simulink model "EEEUI (1)"  (R2024b)
settings: Solver=VariableStepAuto  StartTime=0.0  StopTime=10.0  RelTol=1e-3
libraries: spsBreakerLib x6, spsThreePhaseSourceLib x3, spsGroundLib x2, spsThreePhaseParallelRLCLoadLib x2, spsThreePhaseTransformer12TerminalsLib x2, spsThreePhaseSeriesRLCLoadLib x1, spsThreePhaseVIMeasurementLib x1, spsThreePhaseBreakerLib x1, spsThreePhaseFaultLib x1
settings Model: Creator=praji

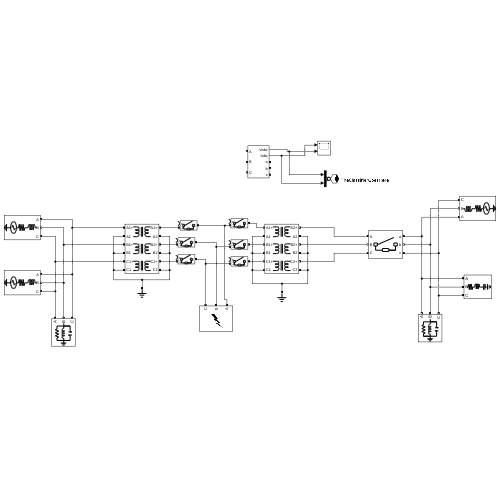
[thumbnail: Simulink's stored preview of the top-level diagram]
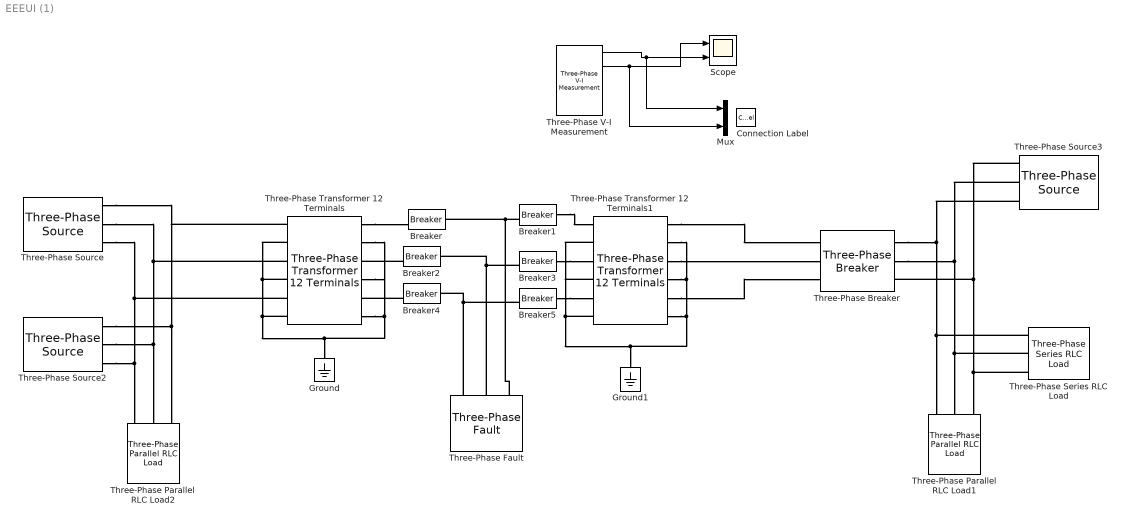
== system EEEUI (1) ==
  Breaker{,1..5} (6 alike) : spsBreakerLib/Breaker  InitialState=0  SwitchingTimes="[1/60  5/60]"  External=on  BreakerResistance=0.01  SnubberResistance=1e6  SnubberCapacitance=inf  Measurements=None  MoreParameters=on  NoBreakLoop=off
  Connection Label : ConnectionLabel  Label=TheClassifierGoesHere
  Ground : spsGroundLib/Ground  LConnTagsString=a
  Ground1 : spsGroundLib/Ground  LConnTagsString=a
  Mux : Mux  Inputs=2
  Scope : Scope  NumInputPorts=2
  Three-Phase Parallel RLC Load1 : spsThreePhaseParallelRLCLoadLib/Three-Phase Parallel RLC Load  LConnTagsString=A|B|C  Configuration=Y (grounded)  NominalVoltage=1000  Vabc=[1e3 1e3 1e3]  Vabcp=[1e3 1e3 1e3]  NominalFrequency=60  UnbalancedPower=off  ActivePower=10e3  InductivePower=100  CapacitivePower=100  Pabc=[10e3 9e3 11e3]  QLabc=[100 90 110]  QCabc=[100 90 110]  Pabcp=[10e3 9e3 11e3]  QLabcp=[100 90 110]  QCabcp=[100 90 110]  Measurements=None  LoadType=constant Z
  Three-Phase Parallel RLC Load2 : spsThreePhaseParallelRLCLoadLib/Three-Phase Parallel RLC Load  LConnTagsString=A|B|C  Configuration=Y (grounded)  NominalVoltage=1000  Vabc=[1e3 1e3 1e3]  Vabcp=[1e3 1e3 1e3]  NominalFrequency=60  UnbalancedPower=off  ActivePower=10e3  InductivePower=100  CapacitivePower=100  Pabc=[10e3 9e3 11e3]  QLabc=[100 90 110]  QCabc=[100 90 110]  Pabcp=[10e3 9e3 11e3]  QLabcp=[100 90 110]  QCabcp=[100 90 110]  Measurements=None  LoadType=constant Z
  Three-Phase Series RLC Load : spsThreePhaseSeriesRLCLoadLib/Three-Phase Series RLC Load  LConnTagsString=A|B|C  Configuration=Y (grounded)  NominalVoltage=1000  Vabc=[1e3 1e3 1e3]  Vabcp=[1e3 1e3 1e3]  NominalFrequency=60  UnbalancedPower=off  ActivePower=10e3  InductivePower=100  CapacitivePower=100  Pabc=[10e3 9e3 11e3]  QLabc=[100 90 110]  QCabc=[100 90 110]  Pabcp=[10e3 9e3 11e3]  QLabcp=[100 90 110]  QCabcp=[100 90 110]  Measurements=None  LoadType=constant Z
  Three-Phase V-I Measurement : spsThreePhaseVIMeasurementLib/Three-Phase V-I Measurement  VoltageMeasurement=phase-to-ground  SetLabelV=off  LabelV=Vabc  Vpu=off  VpuLL=off  CurrentMeasurement=yes  SetLabelI=off  LabelI=Iabc  Ipu=off  Pbase=100e6  Vbase=500e3  OutputType=Complex  PhasorSimulation=off  PSBequivalent=0
  Three-Phase Breaker : spsThreePhaseBreakerLib/Three-Phase Breaker  InitialState=open  SwitchA=on  SwitchB=on  SwitchC=on  SwitchTimes="[1/60  5/60]"  External=off  BreakerResistance=0.01  SnubberResistance=1e6  SnubberCapacitance=inf  Measurements=None
  Three-Phase Fault : spsThreePhaseFaultLib/Three-Phase Fault  InitialStates=0  FaultA=on  FaultB=on  FaultC=on  GroundFault=on  SwitchTimes="[1/60  5/60]"  External=off  SwitchStatus=NaN  FaultResistance=0.001  GroundResistance=0.01  SnubberResistance=1e6  SnubberCapacitance=inf  Measurements=None
  Three-Phase Source : spsThreePhaseSourceLib/Three-Phase Source  InternalConnection=Yg  VoltagePhases=off  Voltage=25e3  PhaseAngle=0  Voltage_phases=[25e3 25e3 25e3]/sqrt(3)  PhaseAngles_phases=[0 -120 +120]  Frequency=60  NonIdealSource=on  SpecifyImpedance=off  Resistance=0.8929  Inductance=16.58e-3  ShortCircuitLevel=100e6  BaseVoltage=25e3  XRratio=7  BusType=swing  Pref=10e3  Qref=0  Prefabc=[10e3, 10e3, 10e3]  Qrefabc=[0, 0, 0]  Qmin=-inf  Qmax=inf
  Three-Phase Source2 : spsThreePhaseSourceLib/Three-Phase Source  InternalConnection=Yg  VoltagePhases=off  Voltage=25e3  PhaseAngle=0  Voltage_phases=[25e3 25e3 25e3]/sqrt(3)  PhaseAngles_phases=[0 -120 +120]  Frequency=60  NonIdealSource=on  SpecifyImpedance=off  Resistance=0.8929  Inductance=16.58e-3  ShortCircuitLevel=100e6  BaseVoltage=25e3  XRratio=7  BusType=swing  Pref=10e3  Qref=0  Prefabc=[10e3, 10e3, 10e3]  Qrefabc=[0, 0, 0]  Qmin=-inf  Qmax=inf
  Three-Phase Source3 : spsThreePhaseSourceLib/Three-Phase Source  InternalConnection=Yg  VoltagePhases=off  Voltage=25e3  PhaseAngle=0  Voltage_phases=[25e3 25e3 25e3]/sqrt(3)  PhaseAngles_phases=[0 -120 +120]  Frequency=60  NonIdealSource=on  SpecifyImpedance=off  Resistance=0.8929  Inductance=16.58e-3  ShortCircuitLevel=100e6  BaseVoltage=25e3  XRratio=7  BusType=swing  Pref=10e3  Qref=0  Prefabc=[10e3, 10e3, 10e3]  Qrefabc=[0, 0, 0]  Qmin=-inf  Qmax=inf
  Three-Phase Transformer 12 Terminals : spsThreePhaseTransformer12TerminalsLib/Three-Phase Transformer 12 Terminals  RatedPower=[ 10e6 60 ]  Winding1="[ 10e3 0.002  0.05 ]"  Winding2=[ 25e3 0.002 0.05]  RmXm=[ 200 200 ]
      settings: LibrarySourceBlock=|
      | sps_lib/Power Grid Elements/Three-Phase Transformer
      | 12 Terminals
  Three-Phase Transformer 12 Terminals1 : spsThreePhaseTransformer12TerminalsLib/Three-Phase Transformer 12 Terminals  RatedPower=[ 10e6 60 ]  Winding1="[ 10e3 0.002  0.05 ]"  Winding2=[ 25e3 0.002 0.05]  RmXm=[ 200 200 ]
      settings: LibrarySourceBlock=|
      | sps_lib/Power Grid Elements/Three-Phase Transformer
      | 12 Terminals
  wires:
  Three-Phase V-I Measurement/1 -> Mux/1, Scope/2
  Three-Phase V-I Measurement/2 -> Mux/2, Scope/1
  connections:
  Three-Phase Source2/RConn1 -- Three-Phase Transformer 12 Terminals/LConn1 -- Three-Phase Source/RConn1 -- Three-Phase Parallel RLC Load2/LConn3
  Three-Phase Source/RConn3 -- Three-Phase Source2/RConn3 -- Three-Phase Parallel RLC Load2/LConn1 -- Three-Phase Transformer 12 Terminals/LConn5
  Three-Phase Source/RConn2 -- Three-Phase Source2/RConn2 -- Three-Phase Parallel RLC Load2/LConn2 -- Three-Phase Transformer 12 Terminals/LConn3
  Three-Phase Transformer 12 Terminals/LConn2 -- Three-Phase Transformer 12 Terminals/LConn4 -- Three-Phase Transformer 12 Terminals/RConn6 -- Three-Phase Transformer 12 Terminals/RConn4 -- Three-Phase Transformer 12 Terminals/RConn2 -- Ground/LConn1 -- Three-Phase Transformer 12 Terminals/LConn6
  Three-Phase Transformer 12 Terminals1/RConn1 -- Three-Phase Breaker/LConn1
  Three-Phase Transformer 12 Terminals1/RConn3 -- Three-Phase Breaker/LConn2
  Three-Phase Transformer 12 Terminals1/RConn5 -- Three-Phase Breaker/LConn3
  Three-Phase Transformer 12 Terminals1/RConn2 -- Three-Phase Transformer 12 Terminals1/RConn4 -- Ground1/LConn1 -- Three-Phase Transformer 12 Terminals1/LConn4 -- Three-Phase Transformer 12 Terminals1/LConn2 -- Three-Phase Transformer 12 Terminals1/LConn6 -- Three-Phase Transformer 12 Terminals1/RConn6
  Three-Phase Source3/RConn1 -- Three-Phase Breaker/RConn1 -- Three-Phase Series RLC Load/LConn1 -- Three-Phase Parallel RLC Load1/LConn1
  Three-Phase Source3/RConn2 -- Three-Phase Breaker/RConn2 -- Three-Phase Series RLC Load/LConn2 -- Three-Phase Parallel RLC Load1/LConn2
  Three-Phase Source3/RConn3 -- Three-Phase Breaker/RConn3 -- Three-Phase Parallel RLC Load1/LConn3 -- Three-Phase Series RLC Load/LConn3
  Three-Phase Transformer 12 Terminals/RConn1 -- Breaker/LConn1
  Three-Phase Fault/LConn1 -- Breaker1/LConn1 -- Breaker/RConn1
  Breaker1/RConn1 -- Three-Phase Transformer 12 Terminals1/LConn1
  Breaker2/LConn1 -- Three-Phase Transformer 12 Terminals/RConn3
  Three-Phase Fault/LConn2 -- Breaker2/RConn1 -- Breaker3/LConn1
  Breaker3/RConn1 -- Three-Phase Transformer 12 Terminals1/LConn3
  Breaker4/LConn1 -- Three-Phase Transformer 12 Terminals/RConn5
  Three-Phase Fault/LConn3 -- Breaker5/LConn1 -- Breaker4/RConn1
  Breaker5/RConn1 -- Three-Phase Transformer 12 Terminals1/LConn5
